simulink model "simulation"  (R2023a)
settings: Solver=VariableStepAuto  StartTime=0.0  StopTime=0.05  RelTol=1e-3
settings Model: Creator=Andre  LastModifiedBy=Andre

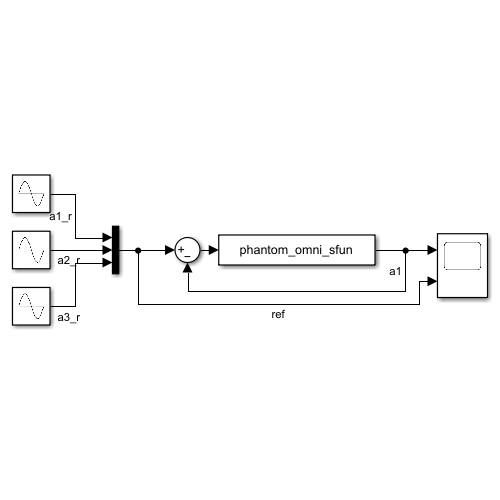
[thumbnail: Simulink's stored preview of the top-level diagram]
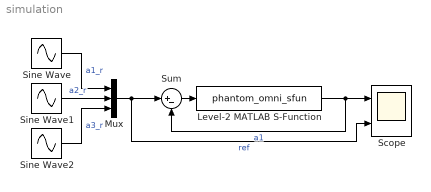
== system simulation ==
  Level-2 MATLAB S-Function : M-S-Function  FunctionName=phantom_omni_sfun  Parameters=0.001, 0, [200;200;200], [50;50;50], [20;20;20], 0.001, 2, 1, 0.5, 0.4, 0.3
  Mux : Mux  Inputs=3
  Scope : Scope  NumInputPorts=2
  Sine Wave : Sin  Amplitude=0.1  Frequency=628.3185  SampleTime=0
  Sine Wave1 : Sin  Amplitude=0.1  Frequency=628.3185  Phase=pi/6  SampleTime=0
  Sine Wave2 : Sin  Amplitude=0.1  Frequency=628.3185  Phase=pi/3  SampleTime=0
  Sum : Sum  Inputs=|+-
  wires:
  Sine Wave/1 -> Mux/1  "a1_r"
  Level-2 MATLAB S-Function/1 -> Sum/2, Scope/1  "a1"
  Sine Wave1/1 -> Mux/2  "a2_r"
  Sine Wave2/1 -> Mux/3  "a3_r"
  Mux/1 -> Scope/2, Sum/1  "ref"
  Sum/1 -> Level-2 MATLAB S-Function/1
